simulink model "escalamiento"  (R2013a)
settings: Solver=ode5  StartTime=0.0  StopTime=10.0  RelTol=1e-3
undefined symbols (not defined in the file or in its folder): National_Instruments, PCI
libraries: rtwinlib x2
settings Model: SimulationMode=external  Creator=u_labelectro  LastModifiedBy=u_labelectro
settings HardwareCC: ProdIntDivRoundTo=Zero  ProdEndianess=LittleEndian  ProdHWDeviceType=Generic->32-bit x86 compatible
settings RTWCC: SystemTargetFile=rtwin.tlc  TemplateMakefile=rtwin.tmf  Description=Real-Time Windows Target  ProcessScript=rtwin_make_rtw_hook  RTWCompilerOptimization=On
settings CodeAppCC: MaxIdLength=95
settings RTWinTargetCC: TargetLibSuffix=_rtwin.lib  TargetPreCompLibLocation=D:\Real Time\toolbox\rtw\targets\rtwin\lib\win64  CodeReplacementLibrary=ANSI_C  RTWinDir=D:/REALTI~1/toolbox/rtw/targets/rtwin  TargetArch=win64

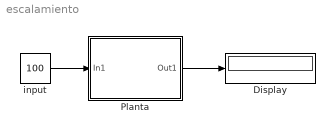
== system escalamiento ==
  Display : Display
  Planta : Subsystem
  input : Constant  Value=100
  wires:
  Planta/1(Out1) -> Display/1
  input/1 -> Planta/1(In1)

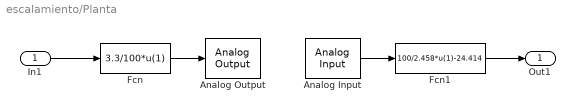
== system escalamiento/Planta ==
  In1 : Inport
  Analog Input : rtwinlib/Analog Input  SampleTime=0.01  MaxMissedTicks=10  ShowMissedTicks=off  YieldWhenWaiting=off  DrvName=National_Instruments/PCI-6229  DrvAddress=4294967295  DrvOptions=[0 0 0 0 0]  Channels=1  RangeMode=1  VoltRange=1  DataType=1
      settings: AttributesFormatString=National Instruments\nPCI-6229 [auto]
  Analog Output : rtwinlib/Analog Output  SampleTime=0.01  MaxMissedTicks=10  ShowMissedTicks=off  YieldWhenWaiting=off  DrvName=National_Instruments/PCI-6229  DrvAddress=4294967295  DrvOptions=[0 0 0 0 0]  Channels=1  RangeMode=1  VoltRange=1  InitialValue=[]  FinalValue=[]
      settings: AttributesFormatString=National Instruments\nPCI-6229 [auto]
  Fcn : Fcn  Expr=3.3/100*u(1)  SampleTime=0.01
  Fcn1 : Fcn  Expr=100/2.458*u(1)-24.414  SampleTime=0.01
  Out1 : Outport
  wires:
  Fcn/1 -> Analog Output/1
  In1/1 -> Fcn/1
  Analog Input/1 -> Fcn1/1
  Fcn1/1 -> Out1/1
